simulink model "lim_grow"  (Simulink 7.9)
settings: Solver=ode45  StartTime=0.0  StopTime=1.0  RelTol=1e-3
values from neighbouring files (symbols this model uses):
  c = 1    [lim_grow_script.m]    (also in predprey.m = 3)
  r = 10    [lim_grow_script.m]    (also in sir.m = 0.55)
settings Model: Creator=Daniel  LastModifiedBy=Daniel

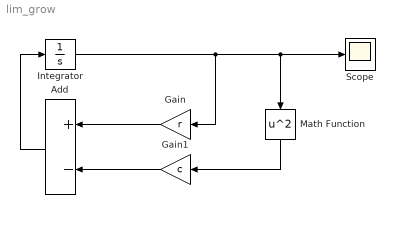
== system lim_grow ==
  Add : Sum  Inputs=+-
  Gain : Gain  Gain=r
  Gain1 : Gain  Gain=c
  Integrator : Integrator  InitialCondition=1
  Math Function : Math  Operator=square  SaturateOnIntegerOverflow=on
  Scope : Scope
  wires:
  Integrator/1 -> Gain/1, Math Function/1, Scope/1
  Math Function/1 -> Gain1/1
  Gain/1 -> Add/1
  Gain1/1 -> Add/2
  Add/1 -> Integrator/1
